simulink model "LabC_FeedbackControl_Robot_DataToMatlab_UseMonitorAndTune"  (R2020a)
settings: Solver=FixedStepDiscrete  StartTime=0.0  StopTime=inf  FixedStep=fSamplingPeriod  RelTol=1e-3  EnableMultiTasking=on
values from neighbouring files (symbols this model uses):
  acc_LSB_per_g = 16384    [GyroAccScaling.mat]
  acc_y_offset = 651.5    [OffsetData.mat]
  acc_z_offset = 170.75    [OffsetData.mat]
  fSamplingPeriod = 0.005    [LabB_ControllerOverSimulator_Discrete_Parameters.m]    (also in LabB_ControllerOverSimulator_Discrete_Parameters_conflict_copy_LAPTOP-FOGVCHE7_2020_11_15.m; LabB_ObserverAndControllerOverSimulator_Discrete_Parameters.m; LabC_6_3.m = 0.2; LabC_6_4.m = 0.067)
  fWheelRadius = 0.0216    [LoadRobotParameters.m]
  gyro_LSB_per_deg = 131    [GyroAccScaling.mat]
  gyro_x_offset = -193.125    [OffsetData.mat]
  K = place(A, B, P)    [LabB_ControllerOverSimulator_Continuous_Parameters.m]    (also in LabB_ControllerOverSimulator_Discrete_Parameters_conflict_copy_LAPTOP-FOGVCHE7_2020_11_15.m; LabB_ObserverAndControllerOverSimulator_Discrete_Parameters.m; LabC_6_6.m; LabC_CompensatorOverRobot_Parameters.m)
  Nud = N    [LabC_6_6.m]    (also in LabC_CompensatorOverRobot_Parameters.m = N_val; LabC_FeedbackControl_Robot_Parameters.m = 0)
  Nxd = 0    [LabC_6_6.m]    (also in LabC_CompensatorOverRobot_Parameters.m; LabC_FeedbackControl_Robot_Parameters.m)
undefined symbols (not defined in the file or in its folder): equ_offset, sigbuilder_block
libraries: MinSegLibrary_M2V3 x4, simulink x2, simulink_extras x1, dspstat3 x1
settings Model: SILPILModeSetting=veronly  ExtModeTrigDuration=2  Creator=pyry  LastModifiedBy=Pyry
settings OptimizationCC: EnhancedBackFolding=on  PassReuseOutputArgsThreshold=0  MaxStackSize=64  OptimizeBlockOrder=speed  DifferentSizesBufferReuse=on  OptimizationCustomize=off
settings DebuggingCC: ParameterTunabilityLossMsg=error
settings HardwareCC: ProdBitPerInt=16  ProdBitPerPointer=16  ProdBitPerSizeT=16  ProdBitPerPtrDiffT=16  ProdLargestAtomicFloat=None  ProdWordSize=8  ProdHWDeviceType=Atmel->AVR  UseEmbeddedCoderFeatures=off
settings SFSimCC: MATLABDynamicMemAlloc=off
settings RTWCC: SystemTargetFile=ert.tlc  HardwareBoard=Arduino Mega 2560  TLCOptions=-aInlineSetEventsForThisBaseRateFcn=TLC_FALSE -aSuppressMultiTaskScheduler=TLC_FALSE -aRateBasedStepFcn=1  TemplateMakefile=ert_default_tmf  GenerateReport=on  Toolchain=Arduino AVR  BuildConfiguration=Faster Runs  LaunchReport=on
settings CodeAppCC: ForceParamTrailComments=on  OperatorAnnotations=on
settings ERTTargetCC: ERTCustomFileBanners=off  SupportContinuousTime=on  SupportNonInlinedSFcns=on  RemoveResetFunc=off  SupportVariableSizeSignals=on  ModelStepFunctionPrototypeControlCompliant=off  ExtModeStaticAllocSize=2048

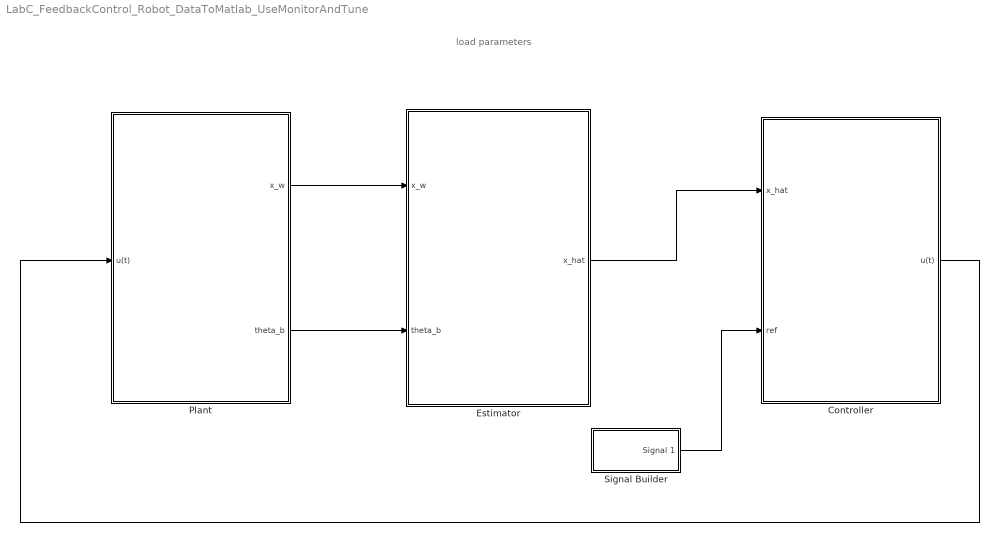
== system LabC_FeedbackControl_Robot_DataToMatlab_UseMonitorAndTune ==
  note: load parameters
  Controller : Subsystem
  Estimator : Subsystem
  Plant : Subsystem
  Signal Builder : Subsystem  Tag=STV Subsys  LoadFcn=sigbuilder_block('load');  StartFcn=sigbuilder_block('start');  StopFcn=sigbuilder_block('stop');  ClipboardFcn=sigbuilder_block('clipboard');  mask(Sigbuilder block){tuvar=[0:10]}
      mask help: Simulink:masks:SigbuilderBlock_MD
      mask init:
      | if ~strcmp(get_param(bdroot(gcbh),'SimulationStatus'),'stopped') tuvar = sigbuilder_block('maskInit'); end
      settings: CopyFcn=sigbuilder_block('copy');  DeleteFcn=sigbuilder_block('delete');  ModelCloseFcn=sigbuilder_block('modelClose');  PreSaveFcn=sigbuilder_block('preSave');  PauseFcn=sigbuilder_block('pause');  ContinueFcn=sigbuilder_block('continue');  NameChangeFcn=sigbuilder_block('namechange');  OpenFcn=sigbuilder_block('open',[437.6 199.2 550.4 400 ]);  CloseFcn=sigbuilder_block('close');
      mask Display: plot(0, 0, 100, 100,[2, 2, 32, 32, 2], [68, 8, 8, 68, 68],[32, 2], [38, 38], [32, 19, 2],[53, 60, 44], [32, 17, 17, 2],[16, 16, 31, 31]);txt = getActiveGroup(gcbh);text(2, 100, txt,'verticalAlignment', 'top');
  wires:
  Plant/1(x_w) -> Estimator/1(x_w)
  Plant/2(theta_b) -> Estimator/2(theta_b)
  Estimator/1(x_hat) -> Controller/1(x_hat)
  Controller/1(u(t)) -> Plant/1(u(t))
  Signal Builder/1(Signal 1) -> Controller/2(ref)

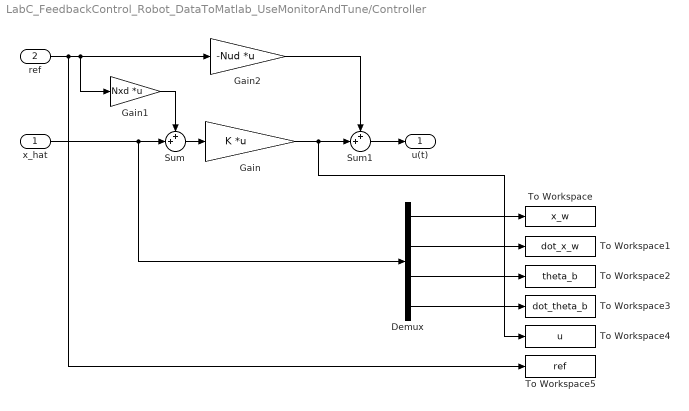
== system LabC_FeedbackControl_Robot_DataToMatlab_UseMonitorAndTune/Controller ==
  x_hat : Inport
  ref : Inport  Port=2
  Demux : Demux
  Gain : Gain  Gain=K  Multiplication=Matrix(K*u)
  Gain1 : Gain  Gain=Nxd  Multiplication=Matrix(K*u)
  Gain2 : Gain  Gain=-Nud  Multiplication=Matrix(K*u)
  Sum : Sum  Inputs=++|
  Sum1 : Sum  Inputs=++|
  To Workspace : ToWorkspace  VariableName=x_w  SaveFormat=Structure With Time  SampleTime=-1
  To Workspace1 : ToWorkspace  VariableName=dot_x_w  SaveFormat=Structure With Time  SampleTime=-1
  To Workspace2 : ToWorkspace  VariableName=theta_b  SaveFormat=Structure With Time  SampleTime=-1
  To Workspace3 : ToWorkspace  VariableName=dot_theta_b  SaveFormat=Structure With Time  SampleTime=-1
  To Workspace4 : ToWorkspace  VariableName=u  SaveFormat=Structure With Time  SampleTime=-1
  To Workspace5 : ToWorkspace  VariableName=ref  SaveFormat=Structure With Time  SampleTime=-1
  u(t) : Outport
  wires:
  x_hat/1 -> Sum/2, Demux/1
  Gain/1 -> To Workspace4/1, Sum1/2
  Demux/1 -> To Workspace/1
  Demux/2 -> To Workspace1/1
  Demux/3 -> To Workspace2/1
  Demux/4 -> To Workspace3/1
  Sum/1 -> Gain/1
  ref/1 -> To Workspace5/1, Gain1/1, Gain2/1
  Gain1/1 -> Sum/1
  Sum1/1 -> u(t)/1
  Gain2/1 -> Sum1/1

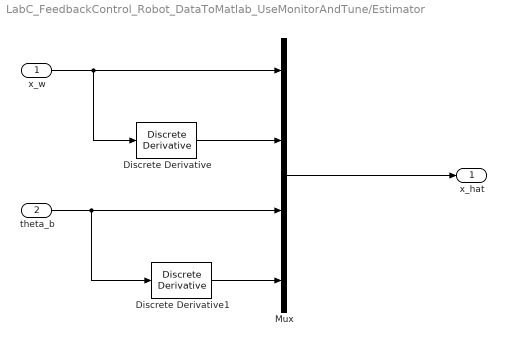
== system LabC_FeedbackControl_Robot_DataToMatlab_UseMonitorAndTune/Estimator ==
  x_w : Inport
  theta_b : Inport  Port=2
  Discrete Derivative : simulink/Discrete/Discrete Derivative  gainval=1.0  ICPrevScaledInput=0.0  OutMin=[]  OutMax=[]  OutDataType=fixdt(1, 16)  OutScaling=2^-10  DoSatur=off
  Discrete Derivative1 : simulink/Discrete/Discrete Derivative  gainval=1.0  ICPrevScaledInput=0.0  OutMin=[]  OutMax=[]  OutDataType=fixdt(1, 16)  OutScaling=2^-10  DoSatur=off
  Mux : Mux
  x_hat : Outport
  wires:
  Mux/1 -> x_hat/1
  Discrete Derivative/1 -> Mux/2
  x_w/1 -> Discrete Derivative/1, Mux/1
  theta_b/1 -> Discrete Derivative1/1, Mux/3
  Discrete Derivative1/1 -> Mux/4

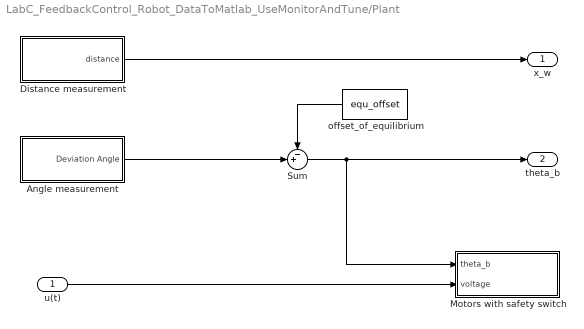
== system LabC_FeedbackControl_Robot_DataToMatlab_UseMonitorAndTune/Plant ==
  u(t) : Inport
  Angle measurement : Subsystem
  Distance measurement : Subsystem
  Motors with safety switch : Subsystem
  Sum : Sum  Inputs=-+|
  offset_of_equilibrium : Constant  Value=equ_offset
  x_w : Outport
  theta_b : Outport  Port=2
  wires:
  Sum/1 -> Motors with safety switch/1("theta_b "), theta_b/1
  Angle measurement/1(Deviation Angle) -> Sum/2
  offset_of_equilibrium/1 -> Sum/1
  Distance measurement/1(distance) -> x_w/1
  u(t)/1 -> Motors with safety switch/2(voltage)

== system LabC_FeedbackControl_Robot_DataToMatlab_UseMonitorAndTune/Signal Builder ==
  Demux : Demux  Tag=STV Demux  Outputs=1
      settings: DisplayOption=none
  FromWs : FromWorkspace  Tag=STV FromWs  VariableName=tuvar
      SigBuilderData=|
      | common.afterFinalStr = 'Extrapolate'
      | common.sampleTime = 0
      | dataSet.timeRange = [0 10]
      | dataSet.name = 'Group 1'
      | sbobj.Groups.Name = 'Group 1'
      | sbobj.Groups.Signals.Name = 'Signal 1'
      | sbobj.Groups.Signals.XData = [0 10]
      | sbobj.Groups.Signals.YData = [0 0]
  Signal 1 : Outport  Tag=STV Outport
  wires:
  Demux/1 -> Signal 1/1
  FromWs/1 -> Demux/1

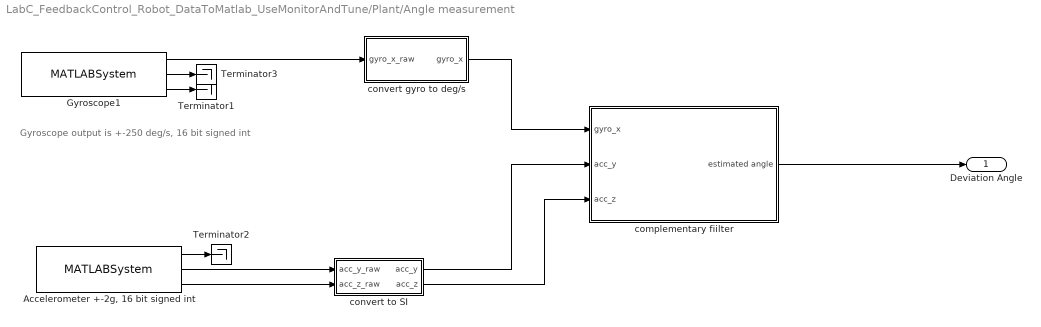
== system LabC_FeedbackControl_Robot_DataToMatlab_UseMonitorAndTune/Plant/Angle measurement ==
  note: Gyroscope output is +-250 deg/s, 16 bit signed int
  "Accelerometer +-2g, 16 bit signed int" : MATLABSystem  System=soMPU6050Accel  SimulateUsing=Code generation
      mask Type: soMPU6050Accel
      mask Display:
      | disp('soMPU6050Accel');
      | port_label('output',1,'xaccel');
      | port_label('output',2,'yaccel');
      | port_label('output',3,'zaccel');
  Gyroscope1 : MATLABSystem  System=soMPU6050Gyro  DLPFmode=0
      mask Type: soMPU6050Gyro
      mask Display:
      | disp('soMPU6050Gyro');
      | port_label('output',1,'xvel');
      | port_label('output',2,'yvel');
      | port_label('output',3,'zvel');
  Terminator1 : Terminator
  Terminator2 : Terminator
  Terminator3 : Terminator
  complementary fiilter : Subsystem
  convert gyro to deg/s : Subsystem
  convert to SI : Subsystem
  Deviation Angle : Outport  VectorParamsAs1DForOutWhenUnconnected=off
  wires:
  complementary fiilter/1(estimated angle) -> Deviation Angle/1
  "Accelerometer +-2g, 16 bit signed int"/2 -> convert to SI/1("acc_y_raw ")
  "Accelerometer +-2g, 16 bit signed int"/3 -> convert to SI/2(acc_z_raw)
  "Accelerometer +-2g, 16 bit signed int"/1 -> Terminator2/1
  convert gyro to deg/s/1(gyro_x) -> complementary fiilter/1(gyro_x)
  convert to SI/1(acc_y) -> complementary fiilter/2(acc_y)
  convert to SI/2(acc_z) -> complementary fiilter/3(acc_z)
  Gyroscope1/3 -> Terminator1/1
  Gyroscope1/2 -> Terminator3/1
  Gyroscope1/1 -> convert gyro to deg/s/1(gyro_x_raw)

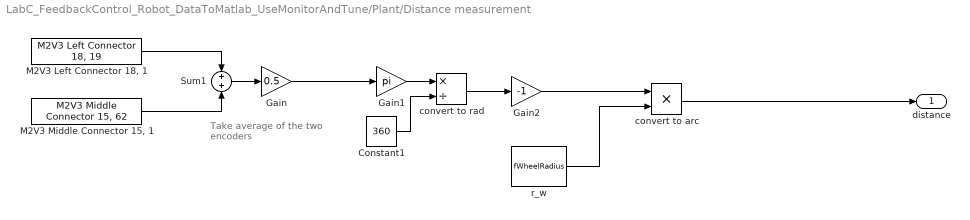
== system LabC_FeedbackControl_Robot_DataToMatlab_UseMonitorAndTune/Plant/Distance measurement ==
  note: Take average of the two encoders
  Constant1 : Constant  Value=360
  Gain : Gain  Gain=0.5
  Gain1 : Gain  Gain=pi
  Gain2 : Gain  Gain=-1
  "M2V3 Left Connector 18, 1" : MinSegLibrary_M2V3/M2V3 Left Connector 18, 19  Encoder=1  PinA=19  PinB=18
      settings: SourceProductName=Rensselaer Arduino Support Package
  "M2V3 Middle Connector 15, 1" : MinSegLibrary_M2V3/M2V3 Middle Connector 15, 62  Encoder=3  PinA=15  PinB=62
      settings: SourceProductName=Rensselaer Arduino Support Package
  Sum1 : Sum
  convert to arc : Product  Inputs=**
  convert to rad : Product  Inputs=*/
  r_w : Constant  Value=fWheelRadius
  distance : Outport  VectorParamsAs1DForOutWhenUnconnected=off
  wires:
  Sum1/1 -> Gain/1
  "M2V3 Left Connector 18, 1"/1 -> Sum1/1
  "M2V3 Middle Connector 15, 1"/1 -> Sum1/2
  Constant1/1 -> convert to rad/2
  Gain1/1 -> convert to rad/1
  r_w/1 -> convert to arc/2
  convert to arc/1 -> distance/1
  convert to rad/1 -> Gain2/1
  Gain2/1 -> convert to arc/1
  Gain/1 -> Gain1/1

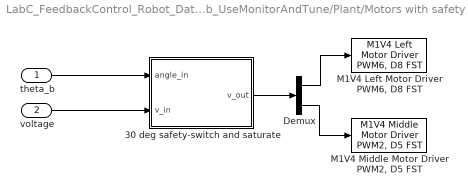
== system LabC_FeedbackControl_Robot_DataToMatlab_UseMonitorAndTune/Plant/Motors with safety switch ==
  "theta_b " : Inport
  voltage : Inport  Port=2
  30 deg safety-switch and saturate : Subsystem
  Demux : Demux  Outputs=2
  "M1V4 Left Motor Driver PWM6, D8 FST" : MinSegLibrary_M2V3/M1V4 Left Motor Driver PWM6, D8 FST  Vsupply=7.2
      settings: SourceProductName=Rensselaer Arduino Support Package
  "M1V4 Middle Motor Driver PWM2, D5 FST" : MinSegLibrary_M2V3/M1V4 Middle Motor Driver PWM2, D5 FST  Vsupply=7.2
      settings: SourceProductName=Rensselaer Arduino Support Package
  wires:
  30 deg safety-switch and saturate/1(v_out) -> Demux/1
  Demux/2 -> "M1V4 Middle Motor Driver PWM2, D5 FST"/1
  Demux/1 -> "M1V4 Left Motor Driver PWM6, D8 FST"/1
  "theta_b "/1 -> 30 deg safety-switch and saturate/1(angle_in)
  voltage/1 -> 30 deg safety-switch and saturate/2(v_in)

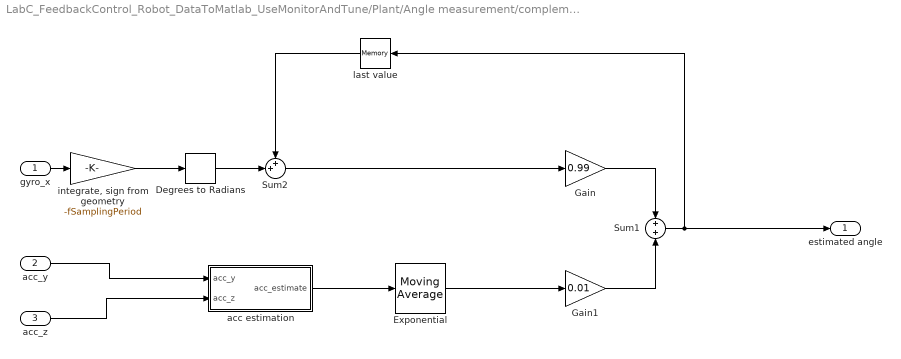
== system LabC_FeedbackControl_Robot_DataToMatlab_UseMonitorAndTune/Plant/Angle measurement/complementary fiilter ==
  gyro_x : Inport
  acc_y : Inport  Port=2
  acc_z : Inport  Port=3
  Degrees to Radians : simulink_extras/Transformations/Degrees to Radians
  Exponential : dspstat3/Moving Average  Method=Exponential weighting  ForgettingFactorPort=off  SpecifyWindowLength=on  WindowLength=4  ForgettingFactor=0.01  SimulateUsing=Code generation
  Gain : Gain  Gain=0.99
  Gain1 : Gain  Gain=0.01
  Sum1 : Sum
  Sum2 : Sum  Inputs=++|
  acc estimation : Subsystem
  "integrate, sign from geometry" : Gain  Gain=-fSamplingPeriod
  last value : Memory
  estimated angle : Outport  VectorParamsAs1DForOutWhenUnconnected=off
  wires:
  acc_y/1 -> acc estimation/1(acc_y)
  acc_z/1 -> acc estimation/2("acc_z ")
  Sum1/1 -> last value/1, estimated angle/1
  Gain/1 -> Sum1/1
  Gain1/1 -> Sum1/2
  last value/1 -> Sum2/1
  "integrate, sign from geometry"/1 -> Degrees to Radians/1
  Degrees to Radians/1 -> Sum2/2
  gyro_x/1 -> "integrate, sign from geometry"/1
  Sum2/1 -> Gain/1
  acc estimation/1(acc_estimate) -> Exponential/1
  Exponential/1 -> Gain1/1

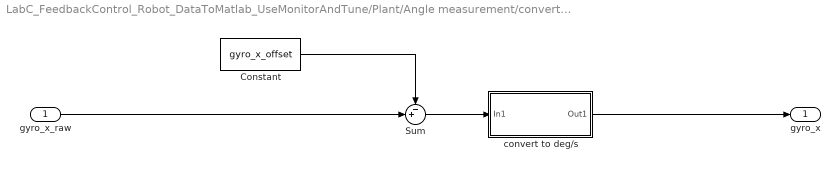
== system LabC_FeedbackControl_Robot_DataToMatlab_UseMonitorAndTune/Plant/Angle measurement/convert gyro to deg//s ==
  gyro_x_raw : Inport
  Constant : Constant  Value=gyro_x_offset
  Sum : Sum  Inputs=-+|
  convert to deg/s : Subsystem
  gyro_x : Outport  VectorParamsAs1DForOutWhenUnconnected=off
  wires:
  gyro_x_raw/1 -> Sum/2
  Sum/1 -> convert to deg/s/1(In1)
  convert to deg/s/1(Out1) -> gyro_x/1
  Constant/1 -> Sum/1

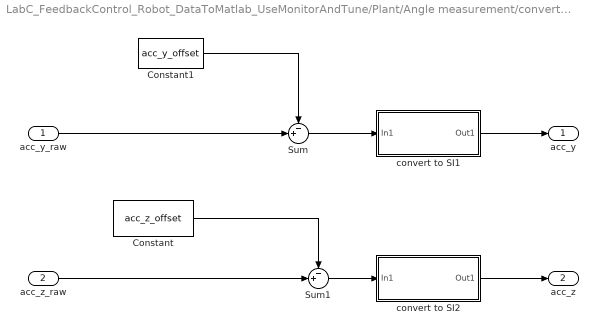
== system LabC_FeedbackControl_Robot_DataToMatlab_UseMonitorAndTune/Plant/Angle measurement/convert to SI ==
  "acc_y_raw " : Inport
  acc_z_raw : Inport  Port=2
  Constant : Constant  Value=acc_z_offset
  Constant1 : Constant  Value=acc_y_offset
  Sum : Sum  Inputs=-+|
  Sum1 : Sum  Inputs=-+|
  convert to SI1 : Subsystem
  convert to SI2 : Subsystem
  acc_y : Outport  VectorParamsAs1DForOutWhenUnconnected=off
  acc_z : Outport  Port=2  VectorParamsAs1DForOutWhenUnconnected=off
  wires:
  convert to SI1/1(Out1) -> acc_y/1
  convert to SI2/1(Out1) -> acc_z/1
  Sum/1 -> convert to SI1/1(In1)
  "acc_y_raw "/1 -> Sum/2
  Sum1/1 -> convert to SI2/1(In1)
  acc_z_raw/1 -> Sum1/2
  Constant/1 -> Sum1/1
  Constant1/1 -> Sum/1

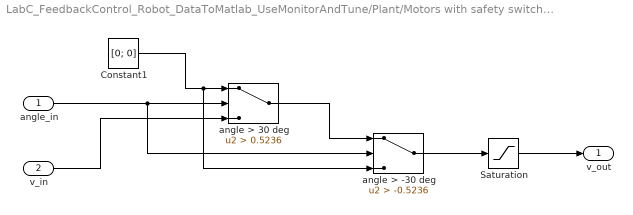
== system LabC_FeedbackControl_Robot_DataToMatlab_UseMonitorAndTune/Plant/Motors with safety switch/30 deg safety-switch and saturate ==
  angle_in : Inport
  v_in : Inport  Port=2
  " angle > -30 deg" : Switch  Criteria=u2 > Threshold  Threshold=-0.5236
  " angle > 30 deg" : Switch  Criteria=u2 > Threshold  Threshold=0.5236
  Constant1 : Constant  Value=[0; 0]  VectorParams1D=off
  Saturation : Saturate  UpperLimit=[7.2; 7.2]  LowerLimit=[-7.2; -7.2]
  v_out : Outport  VectorParamsAs1DForOutWhenUnconnected=off
  wires:
  Constant1/1 -> " angle > -30 deg"/3, " angle > 30 deg"/1
  " angle > 30 deg"/1 -> " angle > -30 deg"/1
  angle_in/1 -> " angle > -30 deg"/2, " angle > 30 deg"/2
  v_in/1 -> " angle > 30 deg"/3
  " angle > -30 deg"/1 -> Saturation/1
  Saturation/1 -> v_out/1

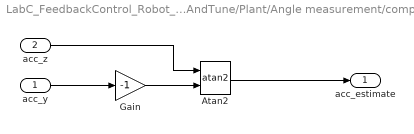
== system LabC_FeedbackControl_Robot_DataToMatlab_UseMonitorAndTune/Plant/Angle measurement/complementary fiilter/acc estimation ==
  acc_y : Inport
  "acc_z " : Inport  Port=2
  Atan2 : Trigonometry  Operator=atan2
  Gain : Gain  Gain=-1
  acc_estimate : Outport  VectorParamsAs1DForOutWhenUnconnected=off
  wires:
  Gain/1 -> Atan2/2
  acc_y/1 -> Gain/1
  "acc_z "/1 -> Atan2/1
  Atan2/1 -> acc_estimate/1

== system LabC_FeedbackControl_Robot_DataToMatlab_UseMonitorAndTune/Plant/Angle measurement/convert gyro to deg//s/convert to deg//s ==
  In1 : Inport
  Divide : Product  Inputs=*/
  Scaling factor from datasheet : Constant  Value=gyro_LSB_per_deg
  Out1 : Outport  VectorParamsAs1DForOutWhenUnconnected=off
  wires:
  Scaling factor from datasheet/1 -> Divide/2
  In1/1 -> Divide/1
  Divide/1 -> Out1/1

== system LabC_FeedbackControl_Robot_DataToMatlab_UseMonitorAndTune/Plant/Angle measurement/convert to SI/convert to SI1 ==
  In1 : Inport
  *9.81 : Gain  Gain=9.81
  Constant : Constant  Value=acc_LSB_per_g
  Divide : Product  Inputs=*/
  Out1 : Outport  VectorParamsAs1DForOutWhenUnconnected=off
  wires:
  Constant/1 -> Divide/2
  In1/1 -> Divide/1
  *9.81/1 -> Out1/1
  Divide/1 -> *9.81/1

== system LabC_FeedbackControl_Robot_DataToMatlab_UseMonitorAndTune/Plant/Angle measurement/convert to SI/convert to SI2 ==
  In1 : Inport
  * - 9.81 : Gain  Gain=-9.81
  Constant : Constant  Value=acc_LSB_per_g
  Divide : Product  Inputs=*/
  Out1 : Outport  VectorParamsAs1DForOutWhenUnconnected=off
  wires:
  Constant/1 -> Divide/2
  In1/1 -> Divide/1
  * - 9.81/1 -> Out1/1
  Divide/1 -> * - 9.81/1
